simulink model "SimscapePumpDataPlant"  (R2026a)
settings: Solver=ode23t  StopTime=simStopTime
libraries: fl_lib x7, nesl_utility x4
settings Model: Creator=rteramot  LastModifiedBy=rteramot

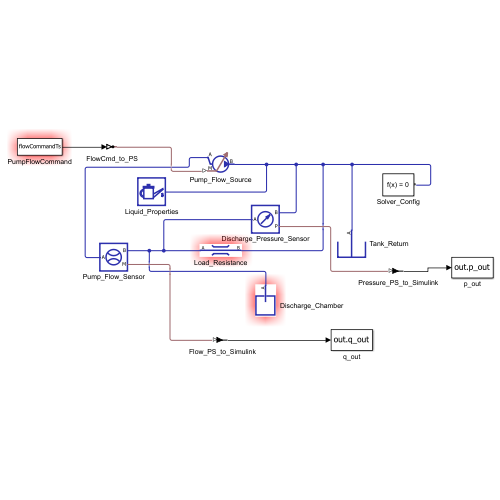
[thumbnail: Simulink's stored preview of the top-level diagram]
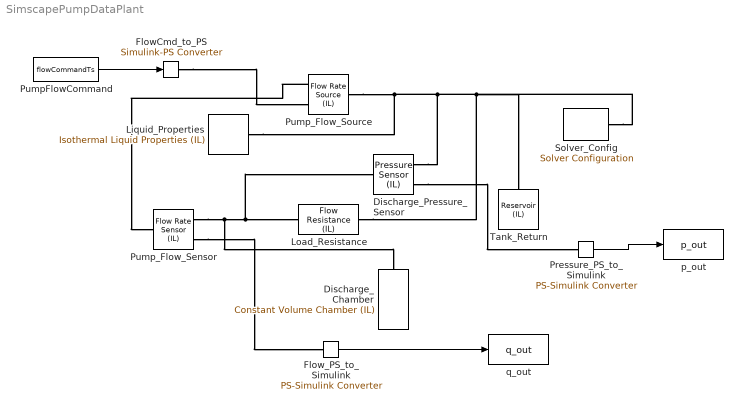
== system SimscapePumpDataPlant ==
  Discharge_Chamber : fl_lib/Isothermal Liquid/Elements/Constant Volume Chamber (IL)  volume=chamberVolume m^3  p_I_specify=on  p_I_priority=High  p_I=101325 Pa  p_I_nominal_specify=off  p_I_nominal_value=1  p_I_nominal_unit=MPa
  Discharge_Pressure_Sensor : fl_lib/Isothermal Liquid/Sensors/Pressure Sensor (IL)  pressure_measure=foundation.enum.pressure_measure.difference
  FlowCmd_to_PS : nesl_utility/Simulink-PS Converter  PhysicalDomain=network_engine_domain  SubClassName=ps_input  LeftPortType=input  RightPortType=output  PseudoPeriodic=off  Frequencies=[]  NoiseDistribution=none  NoiseParameters=[]  Unit=kg/s  AffineConversion=off  FilteringAndDerivatives=filter  SimscapeFilterOrder=1  InputFilterTimeConstant=0.05  UdotUserProvided=0
  Flow_PS_to_Simulink : nesl_utility/PS-Simulink Converter  PhysicalDomain=network_engine_domain  SubClassName=ps_output  LeftPortType=input  RightPortType=output  PseudoPeriodic=off  Frequencies=[]  VectorFormat=inherit  Unit=kg/s  AffineConversion=off
  Liquid_Properties : fl_lib/Isothermal Liquid/Utilities/Isothermal Liquid Properties (IL)  rho_L_atm=998.21 kg/m^3  bulk_modulus_model=foundation.enum.bulk_modulus_model.const  beta_gain=6  beta_L_atm=2.1791e9 Pa  nu_atm=1.0034e-6 m^2/s  p_atm=0.101325 MPa  p_min=1 Pa  properties_range_check=simscape.enum.assert.action.error  air_fraction=0.005  polytropic_index=1.0  rho_g_atm=1.225 kg/m^3  air_dissolution_model=false  p_crit=3 MPa
  Load_Resistance : fl_lib/Isothermal Liquid/Elements/Flow Resistance (IL)  delta_p_nominal=loadPressureDrop Pa  mdot_nominal=nominalMassFlow kg/s  laminar_fraction=0.01
  Pressure_PS_to_Simulink : nesl_utility/PS-Simulink Converter  PhysicalDomain=network_engine_domain  SubClassName=ps_output  LeftPortType=input  RightPortType=output  PseudoPeriodic=off  Frequencies=[]  VectorFormat=inherit  Unit=Pa  AffineConversion=off
  PumpFlowCommand : FromWorkspace  VariableName=flowCommandTs
  Pump_Flow_Sensor : fl_lib/Isothermal Liquid/Sensors/Flow Rate Sensor (IL)  sensor_type=foundation.enum.mass_volumetric_sensor.mass
  Pump_Flow_Source : fl_lib/Isothermal Liquid/Sources/Flow Rate Source (IL)  source_type=foundation.enum.constant_controlled.controlled  flow_type=foundation.enum.mass_volumetric_flow.mass  mass_flow=0 kg/s  volumetric_flow=0 m^3/s
  Solver_Config : nesl_utility/Solver Configuration  PhysicalDomain=network_engine_domain  SubClassName=solver  LeftPortType=input  RightPortType=generic  Tones=[]  Harmonics=[]  SimulateNoise=off  Profile=off  UseLocalSampling=off  EnableSwitchedLinearOptims=on  FrequencyDomain=off  UseCCode=off  RelTol=0.001  AbsTol=0.001  MinStep=1e-09  ToWorkspace=off  RevertToSquareIcSolve=off  NumHomotopyIterations=100  PhasorMode=off  PhasorModeNumHarmonics=1  ConsistencySolver=NEWTON_XTOL_AFTER_FTOL  CanonicalOrdering=CANONICAL  OptimizeIntermediates=OPTIMIZED  IndexReductionMethod=DerivativeReplacement  DoDC=off  ResidualTolerance=1e-09  ConsistencyTolSource=GLOBAL  ConsistencyAbsTol=0.001  ConsistencyRelTol=0.001  ConsistencyTolFactor=0.001  UseLocalSolver=off  LocalSolverChoice=NE_BACKWARD_EULER_ADVANCER  ResolveIndetEquations=on  FunctionEvalNumThread=1  LocalSolverSampleTime=0.001  DoFixedCost=off  MaxNonlinIter=3  MaxModeIter=2  ComputeImpulses=off  ImpulseIterations=2  LinearAlgebra=auto  LinearAlgebraNumThread=0  EquationFormulation=NE_TIME_EF  DelaysMemoryBudget=1024  AutomaticFiltering=on  FilteringTimeConstant=0.001  PartitionStorageMethod=AS_NEEDED  PartitionMemoryBudget=1024  PartitionMethod=ROBUST  MultibodyUseLocalSolver=off  MultibodyLocalSolverChoice=ODE1  MultibodyLocalSolverSampleTime=0.001
  Tank_Return : fl_lib/Isothermal Liquid/Elements/Reservoir (IL)  pressure_input=false  pressure_spec=foundation.enum.pressure_spec.atmospheric  reservoir_pressure=0.101325 MPa
  p_out : ToWorkspace  VariableName=p_out  SaveFormat=Timeseries  SampleTime=-1
  q_out : ToWorkspace  VariableName=q_out  SaveFormat=Timeseries  SampleTime=-1
  wires:
  PumpFlowCommand/1 -> FlowCmd_to_PS/1
  Flow_PS_to_Simulink/1 -> q_out/1
  Pressure_PS_to_Simulink/1 -> p_out/1
  connections:
  Pump_Flow_Source/LConn1 -- Pump_Flow_Sensor/LConn1
  Pump_Flow_Sensor/RConn1 -- Discharge_Pressure_Sensor/LConn1 -- Load_Resistance/LConn1 -- Discharge_Chamber/LConn1
  Discharge_Pressure_Sensor/RConn1 -- Solver_Config/RConn1 -- Tank_Return/LConn1 -- Load_Resistance/RConn1 -- Pump_Flow_Source/RConn1 -- Liquid_Properties/RConn1
  FlowCmd_to_PS/RConn1 -- Pump_Flow_Source/LConn2
  Pump_Flow_Sensor/RConn2 -- Flow_PS_to_Simulink/LConn1
  Discharge_Pressure_Sensor/RConn2 -- Pressure_PS_to_Simulink/LConn1
